simulink model "A2"  (R2017a)
settings: Solver=ode45  StartTime=0.0  StopTime=0.25  MaxStep=1e-4  RelTol=1e-3
libraries: powerlib x15
settings Model: Creator=Amir Reza  LastModifiedBy=Amir Reza

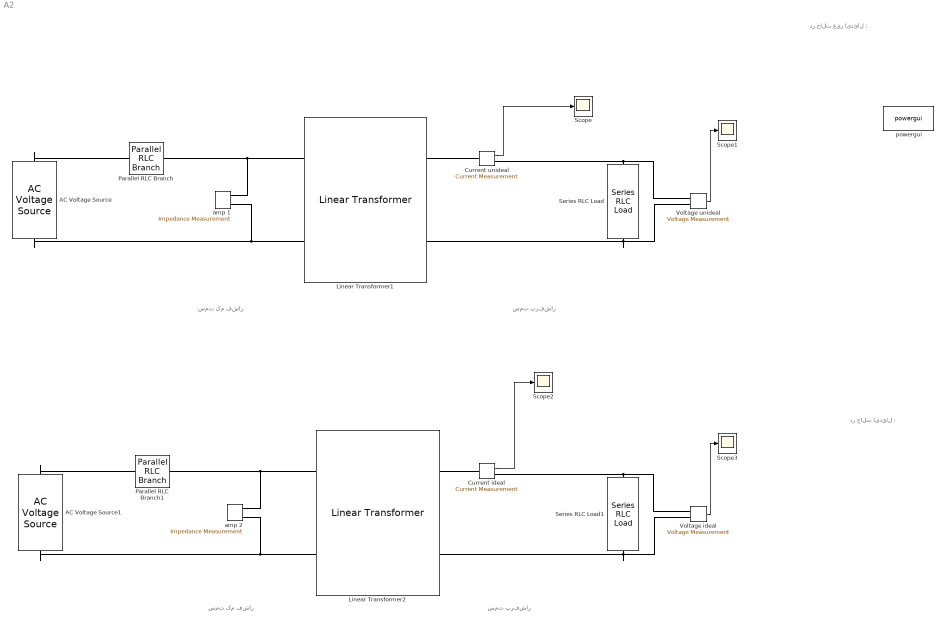
== system A2 ==
  note: سمت پرفشار
  note: در حالت ایدئال :
  note: در حالت غیر ایدئال :
  note: سمت کم فشار
  note: سمت پرفشار
  note: سمت کم فشار
  AC Voltage Source : powerlib/Electrical Sources/AC Voltage Source  Amplitude=240  Phase=0  Frequency=50  SampleTime=0  Measurements=None  BusType=swing  Pref=10e3  Qref=0  Qmin=-inf  Qmax=+inf
  AC Voltage Source1 : powerlib/Electrical Sources/AC Voltage Source  Amplitude=240  Phase=0  Frequency=50  SampleTime=0  Measurements=None  BusType=swing  Pref=10e3  Qref=0  Qmin=-inf  Qmax=+inf
  Current ideal : powerlib/Measurements/Current Measurement  PhasorSimulation=off  OutputType=Complex  PSBequivalent=0
  Current unideal : powerlib/Measurements/Current Measurement  PhasorSimulation=off  OutputType=Complex  PSBequivalent=0
  Linear Transformer1 : powerlib/Elements/Linear Transformer  UNITS=SI  NominalPower=[75e3 50 ]  winding1=[240 6e-3 7.57e-5]  winding2=[2400 0.23 9.74e-3]  ThreeWindings=off  winding3=[3.15e+05 1.0502e+06 354.69]  RmLm=[25 3.97e-2]  Measurements=None  DataType=on
  Linear Transformer2 : powerlib/Elements/Linear Transformer  UNITS=SI  NominalPower=[75e3 50 ]  winding1=[240 0 0]  winding2=[2400 0 0]  ThreeWindings=off  winding3=[3.15e+05 1.0502e+06 354.69]  RmLm=[25 3.97e-2]  Measurements=None  DataType=on
  Parallel RLC Branch : powerlib/Elements/Parallel RLC Branch  LConnTagsString=a  RConnTagsString=__new0  BranchType=R  Resistance=1  Inductance=1e-3  SetiL0=off  InitialCurrent=0  Capacitance=1e-6  Setx0=off  InitialVoltage=0  Measurements=None
  Parallel RLC Branch1 : powerlib/Elements/Parallel RLC Branch  LConnTagsString=a  RConnTagsString=__new0  BranchType=R  Resistance=1  Inductance=1e-3  SetiL0=off  InitialCurrent=0  Capacitance=1e-6  Setx0=off  InitialVoltage=0  Measurements=None
  Scope{,1..3} (4 alike) : Scope
  Series RLC Load : powerlib/Elements/Series RLC Load  LConnTagsString=a  RConnTagsString=__new0  NominalVoltage=2400  NominalFrequency=50  ActivePower=60e3  InductivePower=48  CapacitivePower=0  Setx0=off  InitialVoltage=0  SetiL0=off  InitialCurrent=0  Measurements=None  LoadType=constant Z
  Series RLC Load1 : powerlib/Elements/Series RLC Load  LConnTagsString=a  RConnTagsString=__new0  NominalVoltage=2400  NominalFrequency=50  ActivePower=60e3  InductivePower=48  CapacitivePower=0  Setx0=off  InitialVoltage=0  SetiL0=off  InitialCurrent=0  Measurements=None  LoadType=constant Z
  Voltage ideal : powerlib/Measurements/Voltage Measurement  PhasorSimulation=off  OutputType=Complex  PSBequivalent=0
  "Voltage unideal " : powerlib/Measurements/Voltage Measurement  PhasorSimulation=off  OutputType=Complex  PSBequivalent=0
  "amp 1 " : powerlib/Measurements/Impedance Measurement  LConnTagsString=+|-  Factor=1
      settings: SourceProductName=Simscape Power Systems  SourceProductBaseCode=PS
  amp 2 : powerlib/Measurements/Impedance Measurement  LConnTagsString=+|-  Factor=1
      settings: SourceProductName=Simscape Power Systems  SourceProductBaseCode=PS
  powergui : powerlib/powergui  Priority=1  SimulationMode=Continuous  SampleTime=50e-6  frequency=50  Iterations=50  frequencyindice=50  Pbase=100e6  ErrMax=1e-4  UnitsV=kV  UnitsW=MW  buscounter=0  FunctionMessages=off  echomessages=off  EnableUseOfTLC=off  CurrentSourceSwitches=off  DisableSnubberDevices=off  DisableRonSwitches=off  DisableVfSwitches=off  DisplayEquations=off  SolverType=Tustin/Backward Euler (TBE)  Interpol=off  ExternalGateDelay=off  methode=off  Ts=100  x0status=blocks  SPID=on  SwTol=0  HookPort=off  RestoreLinks=warning  ResistiveCurrentMeasurement=off  Frange=[0:50]  Ylog=off  Xlog=off  ShowGrid=off  save=off  variable=ZData  structure=0  ZoomFFT=off  StartTime=0.0  cycles=1  DisplayStyle=1  fundamental=60  FreqAxis=off  MaxFrequency=1000  frequencyindicesteady=50  RmsSteady=1  display=off
  wires:
  "Voltage unideal "/1 -> Scope1/1
  Voltage ideal/1 -> Scope3/1
  Current ideal/1 -> Scope2/1
  Current unideal/1 -> Scope/1
  connections:
  Series RLC Load/RConn1 -- Linear Transformer1/RConn2 -- "Voltage unideal "/LConn2
  "amp 1 "/LConn1 -- Linear Transformer1/LConn1 -- Parallel RLC Branch/RConn1
  AC Voltage Source/LConn1 -- Linear Transformer1/LConn2 -- "amp 1 "/LConn2
  Linear Transformer1/RConn1 -- Current unideal/LConn1
  Current unideal/RConn1 -- Series RLC Load/LConn1 -- "Voltage unideal "/LConn1
  AC Voltage Source/RConn1 -- Parallel RLC Branch/LConn1
  AC Voltage Source1/LConn1 -- Linear Transformer2/LConn2 -- amp 2/LConn2
  AC Voltage Source1/RConn1 -- Parallel RLC Branch1/LConn1
  Parallel RLC Branch1/RConn1 -- Linear Transformer2/LConn1 -- amp 2/LConn1
  Voltage ideal/LConn2 -- Linear Transformer2/RConn2 -- Series RLC Load1/RConn1
  Voltage ideal/LConn1 -- Series RLC Load1/LConn1 -- Current ideal/RConn1
  Linear Transformer2/RConn1 -- Current ideal/LConn1
